simulink model "Offline_Preprocessing_ECGandSCG3D"  (R2019a)
settings: Solver=FixedStepDiscrete  StartTime=0.0  StopTime=param_sim_time  FixedStep=1/fs  MaxStep=1/fs  RelTol=1e-3
undefined symbols (not defined in the file): fdesignblkfcn, fs, gcbh
(part 2 of 3)

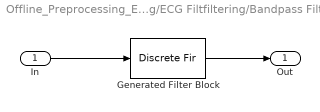
== system Offline_Preprocessing_ECGandSCG3D/ECG Preprocessing/ECG Filtfiltering/Bandpass Filter 2 ==
  In : Inport
  Generated Filter Block : DiscreteFir  Tag=BlockMethodSubSystem  Coefficients=[-0.0116406344063622168 0.00576809638741981705 0.00412102174232116189 0.00269274783173200846 0.00147079622405396279 0.000491631581443595714 -0.000279527338118035207 -0.000824440163218089286 -0.0011931089442172027 -0.00137786624889967881 -0.00143680610402490035 -0.0013658599370285178 -0.00122537593751419899 -0.00100892957375263437 -0.000775151304297802199 -0.000510774577038271629 -0.00027121264178328261 -3.21617788413223332e-05 0.000150365289888468659 0.000323517566100257545 0.000410189273670719806 0.00049803134316846881 0.000505564927906845124 0.000475157220458219745 0.000425303838401711043 0.000342667518480603561 0.000218386639681151032 9.32202317054566659e-05 -3.87356123631495824e-05 -0.000159506396561761091 -0.00028910293766154678 -0.000397731647781897693 -0.0004962822578398942 -0.000556158228593433418 -0.000601142291741041737 -0.00061032042524469636 -0.000610411153005745166 -0.000575325879602293574 -0.000532487836056453126 -0.000454667284566329447 -0.000377559062145994481 -0.000278724916437145948 -0.000187745128628987248 -9.74324644924737249e-05 -1.60738650468866817e-05 5.9764814736124397e-05 0.000109987183421211138 0.000157422257216391359 0.000176177967607079114 0.00018056911694317411 0.000152238854462556986 0.000116164138403226577 5.20308008613596523e-05 -1.73239994344202841e-05 -0.000108419462697777885 -0.000192758346105910763 -0.000288114649125117278 -0.00036987488099304508 -0.00045763639443521624 -0.000524326642655037131 -0.00058632464066331845 -0.000620766605119459774 -0.00064268165693386059 -0.000638078579740596064 -0.000620092611563771018 -0.000572834914300220099 -0.000519984983498502501 -0.000440578049522327708 -0.000362776463167686913 -0.000271958458209525106 -0.000191413582727147438 -0.000103296930882701768 -3.48626201441531308e-05 3.13573430135057063e-05 7.15775158072421563e-05 0.000103833267199419932 0.000103391792586697215 9.08011246543508066e-05 4.6939312636908731e-05 -5.62656538495055758e-06 -8.48056019403329447e-05 -0.000169065203230319219 -0.000271297028825072742 -0.000368012740422246978 -0.00047280159332896074 -0.000559355242459418089 -0.000646838198869518349 -0.000706291730566098452 -0.000756959227202433707 -0.000776213928397353342 -0.00078351986501341668 -0.000757139075089350091 -0.000720571226219025862 -0.000653100073902892694 -0.000578446102546691446 -0.000480516490167021831 -0.000386704679715342906 -0.000280864569862355681 -0.000188982750800533589 -9.63843912055121349e-05 -2.87701546104728728e-05 2.98969073572342287e-05 5.62378466815432326e-05 6.85710121285463409e-05 4.34826849005191807e-05 5.4043371536319218e-06 -6.74672227912870293e-05 -0.000148541085202819056 -0.000256137309555011863 -0.000364360021022150371 -0.000487775998109139797 -0.000597948333952508931 -0.000711693120677205429 -0.000801648264494816964 -0.000884116668799860006 -0.000934017261241329444 -0.000969583957585701262 -0.000967017051073068221 -0.000947278381884976081 -0.000890870622043564431 -0.000821286176068025675 -0.000720694584109535935 -0.000616440121337090766 -0.000492831386257134782 -0.000379545392445496468 -0.000259339184515096702 -0.00016178941864374366 -7.10042565194822506e-05 -1.3392901324712006e-05 2.78153978735731083e-05 2.90754142912783009e-05 1.10946459254170071e-05 -4.76087551916030277e-05 -0.000122756950540332116 -0.000231389766655416482 -0.000347967152363855281 -0.00048791369964742981 -0.000622520837549468686 -0.000765575302446700606 -0.000888640186329310924 -0.00100616465864617095 -0.00109050986367765362 -0.00115914378470589191 -0.00118627235524722263 -0.00119192917236833271 -0.00115382032932690066 -0.00109540150637619203 -0.000999331912807106815 -0.000890174731215546966 -0.000753722389353950195 -0.000618155844393425413 -0.000470259752504975648 -0.000339360741956546905 -0.000212343108328122768 -0.000116871493706854207 -3.89508706146440148e-05 -3.8656480634054885e-06 6.81299165694246311e-06 -2.87912369563211173e-05 -8.92169780942544954e-05 -0.000192214698281994306 -0.000312039737549282131 -0.000463894441742667904 ...(+18228 chars)]  InputProcessing=Columns as channels (frame based)
  Out : Outport
  wires:
  Generated Filter Block/1 -> Out/1
  In/1 -> Generated Filter Block/1

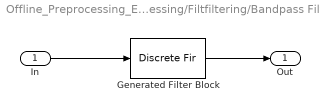
== system Offline_Preprocessing_ECGandSCG3D/SCG Preprocessing/Filtfiltering/Bandpass Filter 1 ==
  In : Inport
  Generated Filter Block : DiscreteFir  Tag=BlockMethodSubSystem  Coefficients=[-0.0141280809748905063 0.00296128789229214984 0.00257104999710791246 0.00216178345802759894 0.00175552729414368662 0.00135185618919181523 0.000971465225508613001 0.000611761661220511233 0.000291406420521247295 4.82187739942602223e-06 -0.000231481095028285982 -0.000426883300566133911 -0.000566810793415535585 -0.000665092291782777567 -0.000708283395739302962 -0.000716103852974445468 -0.000671547633475147107 -0.000615106494933575706 -0.000488109909377568499 -0.00039023478995398736 -0.000258144491787605512 -0.000103777427082112073 3.69273719203651318e-05 0.000160217379967238921 0.00026671934668279218 0.000355855181711751956 0.000424443549910188608 0.000465107287062506772 0.000475941357662008208 0.000454361654694538514 0.000405500722306972525 0.000332653752196094069 0.000244041476717740333 0.00014586724510358938 4.31958982818371473e-05 -5.15123314383907072e-05 -0.000142923677775262659 -0.000215518203590017721 -0.000261730266501079833 -0.000295405514048382306 -0.000292589040735063977 -0.000262673662663612945 -0.000200239042161716452 -0.000119059290944021831 -1.21322536876904141e-05 0.000106963831734455464 0.000240299074014294067 0.000369441485673960984 0.000494924114257010855 0.000600074273648200374 0.000689180050721825352 0.000747556211879633545 0.00078370018100067107 0.000783037479294822897 0.000758170640681550198 0.000702221229410838685 0.000622349141820060375 0.000526336913415630103 0.0004221607579704377 0.000311595034642016266 0.000210279303290487191 0.000121163221325864406 5.51843108116331638e-05 1.14901317572538297e-05 4.63268984994893995e-07 1.97600364123372979e-05 7.52585257249131778e-05 0.000158650819102969243 0.000270390241192615052 0.000399318062573159396 0.000542643635713867603 0.000686965575031424705 0.000829095406210478628 0.000950782043587857992 0.0010553151063333998 0.00112430123884551918 0.0011622562756376225 0.00116100403898215625 0.00112659092458895771 0.00105319818945402016 0.000953344560012619677 0.00082717997461351396 0.000689621114973434923 0.000542798204792277472 0.000403935329663575315 0.000276677120819600331 0.000176948147897282651 0.000104790831399961468 7.17507496432005787e-05 7.47958920750239897e-05 0.000118980916023992203 0.000199000478147194973 0.00031203632149321564 0.000446906185270594392 0.000599958367208587584 0.000753866459386066251 0.000903768587261084486 0.00103429112272444314 0.00114049954630186107 0.00120812081357754564 0.0012369177975026964 0.00121863837734640518 0.00115823236504881272 0.00105257319614870948 0.000912433904619806835 0.000740597166721836814 0.00055288455397877953 0.000354055164106342052 0.000163199294344704149 -1.50951637483461715e-05 -0.000162513118388463509 -0.000275080946577500873 -0.000341943188723371067 -0.000363442033376477208 -0.000334152024712770779 -0.000262311282575287269 -0.000148736623332618167 -6.29165138524290235e-06 0.000158313981566033518 0.000327534481367998398 0.000492510275335981268 0.000636058676656055949 0.000750308535347661912 0.000820834153970441752 0.000843500867080388891 0.000811058974000753233 0.000725579145441402479 0.000586861203976198065 0.000405054868711677424 0.000184940546124497812 -5.59002280569632914e-05 -0.000308204861095151203 -0.000553436858002373175 -0.000780717962187633605 -0.000972296884021750865 -0.00112115970011063097 -0.00121428591472380436 -0.00125044236292902802 -0.00122449203339277529 -0.00114390543564520802 -0.00101139494448911071 -0.000841431774385828155 -0.000642541957157681184 -0.000434750691331326627 -0.000229897013949618978 -4.7878360165821976e-05 9.95394904554497417e-05 0.000197094197447362368 0.000237758271413071945 0.000212546719104122692 0.00012393084974939364 -2.84437637916700597e-05 -0.000234134053639619213 -0.000484592671067755887 -0.00076205183701505072 -0.00105285099253674998 -0.00133585896082410137 -0.00159595443115483765 -0.00181366900494322678 -0.00197783075368639615 -0.00207501327682031202 -0.00210124750065169945 -0.00205143676620883446 -0.00193252830137261369 -0.00174852769809145589 -0.00151582984003622787 ...(+13691 chars)]  InputProcessing=Columns as channels (frame based)
  Out : Outport
  wires:
  Generated Filter Block/1 -> Out/1
  In/1 -> Generated Filter Block/1
